simulink model "tutorial22_root_locus"  (R2025a)
settings: Solver=VariableStepAuto  StartTime=0.0  StopTime=10.0  RelTol=1e-3
settings Model: Creator=xing2  LastModifiedBy=xing2

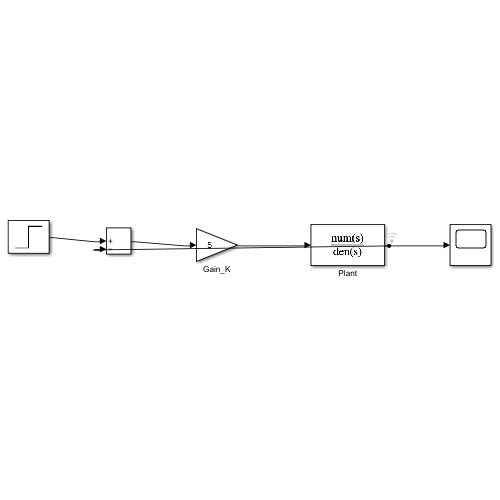
[thumbnail: Simulink's stored preview of the top-level diagram]
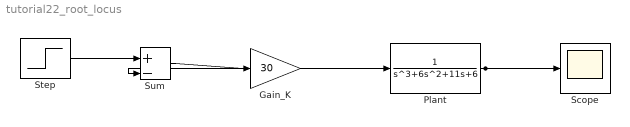
== system tutorial22_root_locus ==
  Gain_K : Gain  Gain=30
  Plant : TransferFcn  Denominator=[1 6 11 6]
  Scope : Scope
  Step : Step  Time=0.5  SampleTime=0
  Sum : Sum  Inputs=|+-
  wires:
  Step/1 -> Sum/1
  Sum/1 -> Gain_K/1
  Gain_K/1 -> Plant/1
  Plant/1 -> Scope/1, Sum/2
